simulink model "A1_10_Parameter_Test"  (Simulink 7.4)
settings: Solver=FixedStepDiscrete  StartTime=0.0  StopTime=10.0  RelTol=1e-3
undefined symbols (not defined in the file): dend, Kp, numd, tau
libraries: DCmotor_library x1
settings Model: Creator=Patrick  LastModifiedBy=ma
settings OptimizationCC: ExpressionDepthLimit=128
settings DebuggingCC: FcnCallInpInsideContextMsg=Enable All  StrictBusMsg=ErrorLevel1
settings CodeAppCC: CustomSymbolStrType=$N$R$M_T
settings GRTTargetCC: CombineOutputUpdateFcns=on

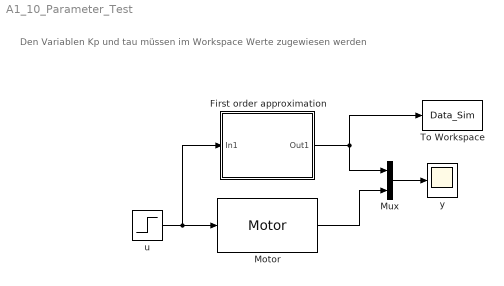
== system A1_10_Parameter_Test ==
  note: Den Variablen
      | Kp und tau
      | müssen im Workspace
      | Werte zugewiesen werden
  First order approximation : Subsystem  mask(DiscretizedTransferFcn){Numerator=[Kp], Denominator=[tau 1], AbsTol=auto, SampleTime=0.01, method=tustin, Wc=1}
      mask prompts: Numerator "Numerator (enter in s-domain:)"; Denominator "Denominator (enter in s-domain:)"; AbsTol "Absolute tolerance:"; SampleTime "Sample time:"; Wc "Critical Frequency (Hz):"
      mask help: Continuous mask uses c2d to transform parameters onto the Discrete Transfer function block inside.
      mask init:
      | st=SampleTime;
      | if length(st)>1
      |     st=SampleTime(1);
      | end
      | if(st>0)
      |     [numd,dend] = sldiscutil('disctransferfcn',{st,method,Wc,Numerator,Denominator});
      | end	
      | s = get_param(gcb,'maskvalues');
      | nums = s{1};
      | dens = s{2};
      | %numc = eval(nums);
      | %denc = eval(dens);
      | sldiscutil('inittfmask', st);
      | if(st==0)
      | set_param([gcb '/Transfer Fcn'], 'AbsoluteTolerance', AbsTol);
      | end
      mask StyleString: edit,edit,edit,edit,popup(zoh|foh|tustin|prewarp|matched),edit
      mask CallbackString: ||||hidecrit|
      mask Display:
      | dpoly(nums,dens)
      | text( 0.5, 1.0, method, 'verticalAlignment','top')
  Motor : DCmotor_library/Motor  motoridinput=8  name_signal=Velocity  ts=10
  Mux : Mux  Inputs=2
  To Workspace : ToWorkspace  VariableName=Data_Sim  SampleTime=-1  SaveFormat=Structure With Time
  u : Step  After=6  SampleTime=0.01
  y : Scope
      settings: YMin=-10  YMax=140
  wires:
  u/1 -> First order approximation/1(In1), Motor/1
  Motor/1 -> Mux/2
  Mux/1 -> y/1
  First order approximation/1(Out1) -> Mux/1, To Workspace/1

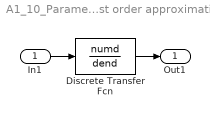
== system A1_10_Parameter_Test/First order approximation ==
  In1 : Inport
  Discrete Transfer Fcn : DiscreteTransferFcn  Numerator=numd  Denominator=dend  SampleTime=SampleTime
  Out1 : Outport
  wires:
  In1/1 -> Discrete Transfer Fcn/1
  Discrete Transfer Fcn/1 -> Out1/1
